simulink model "PARTEB"  (R2020b)
settings: Solver=VariableStepAuto  StartTime=0.0  StopTime=20  RelTol=1e-3
libraries: pid_lib x1
settings Model: Creator=User  LastModifiedBy=angello

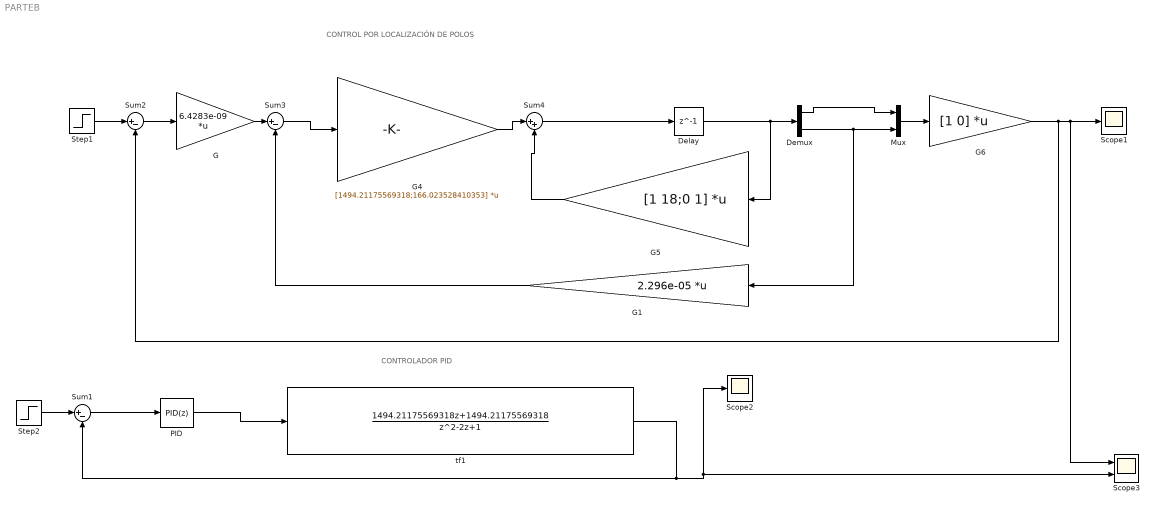
== system PARTEB ==
  note: CONTROL POR LOCALIZACIÓN DE POLOS
  note: CONTROLADOR PID
  Delay : Delay  DelayLength=1  InitialCondition=0
  Demux : Demux  Outputs=2
  G : Gain  Gain=6.4283e-09  Multiplication=Matrix(K*u)
  G1 : Gain  Gain=2.296e-05  Multiplication=Matrix(K*u)
  G4 : Gain  Gain=[1494.21175569318;166.023528410353]  Multiplication=Matrix(K*u)
  G5 : Gain  Gain=[1 18;0 1]  Multiplication=Matrix(K*u)
  G6 : Gain  Gain=[1 0]  Multiplication=Matrix(K*u)
  Mux : Mux  Inputs=2
  PID : pid_lib/PID Controller  Controller=PID  Form=Parallel  TimeDomain=Discrete-time  UseExternalTs=off  SampleTime=-1  IntegratorMethod=Forward Euler  FilterMethod=Forward Euler  ControllerParametersSource=internal  P=4.3719  I=1.7458  D=10.8844  UseFilter=on  N=100  TunerSelectOption=Transfer Function Based (PID Tuner App)  InitialConditionSource=internal  InitialConditionForIntegrator=0  InitialConditionForFilter=0  DifferentiatorICPrevScaledInput=0  ExternalReset=none  TrackingMode=off  Kt=1  LimitOutput=off  SatLimitsSource=internal  UpperSaturationLimit=inf  LowerSaturationLimit=-inf  LinearizeAsGain=off  AntiWindupMode=none  Kb=1  POutMin=[]  POutMax=[]  IOutMin=[]  IOutMax=[]  DOutMin=[]  DOutMax=[]  NOutMin=[]  NOutMax=[]  SumOutMin=[]  SumOutMax=[]  SaturationOutMin=[]  SaturationOutMax=[]  PParamMin=[]  PParamMax=[]  IParamMin=[]  IParamMax=[]  DParamMin=[]  DParamMax=[]  NParamMin=[]  NParamMax=[]  KbParamMin=[]  KbParamMax=[]  KtParamMin=[]  KtParamMax=[]  KbOutMin=[]  KbOutMax=[]  KtOutMin=[]  KtOutMax=[]  IntegratorOutMin=[]  IntegratorOutMax=[]  FilterOutMin=[]  FilterOutMax=[]  SumI1OutMin=[]  SumI1OutMax=[]  SumI2OutMin=[]  SumI2OutMax=[]  SumI3OutMin=[]  SumI3OutMax=[]  SumI4OutMin=[]  SumI4OutMax=[]  SumDOutMin=[]  SumDOutMax=[]  DifferentiatorOutMin=[]  DifferentiatorOutMax=[]  FilterDiffOutCoefMin=[]  FilterDiffOutCoefMax=[]  ReciprocalOutMin=[]  ReciprocalOutMax=[]  SumDenOutMin=[]  SumDenOutMax=[]  SumNumOutMin=[]  SumNumOutMax=[]  DivideOutMin=[]  DivideOutMax=[]  UdiffTsProdOutMin=[]  UdiffTsProdOutMax=[]  NTsProdOutMin=[]  NTsProdOutMax=[]  UintegralTsProdOutMin=[]  UintegralTsProdOutMax=[]  UngainTsProdOutMin=[]  UngainTsProdOutMax=[]  IntegratorContinuousStateAttributes=''  IntegratorStateMustResolveToSignalObject=off  IntegratorRTWStateStorageClass=Auto  FilterContinuousStateAttributes=''  FilterStateMustResolveToSignalObject=off  FilterRTWStateStorageClass=Auto  ParallelPVariant=InternalParameters  IdealPVariant=Disabled  IVariant=InternalParameters  DVariant=InternalParameters  IntegratorVariant=Discrete  SatVariant=Disabled  AWVariant=Passthrough  PCopyVariant=Disabled  TRVariant=Disabled  FdbkBlocksVariant=Forward  IdealPFdbkVariant=Disabled  SatFdbkVariant=Disabled  DerivativeFilterVariant=ForwardEulerFilter  NVariant=InternalParameters  NCopyVariant=Disabled  FilterICVariant=InternalICsFilter  IntegratorICVariant=InternalICs  ExternalResetVariant=Disabled  TRSumVariant=Passthrough  SumFdbkVariant=Disabled  SumVariant=Sum_PID  TsampFilterVariant=InternalTs  TsampNgainVariant=Passthrough  TsampIntegralVariant=Passthrough  ExternalSaturationOutDataTypeStr=Inherit: Same as second input
  Scope1 : Scope
  Scope2 : Scope
  Scope3 : Scope  NumInputPorts=2
  Step1 : Step  Time=0  SampleTime=0.01
  Step2 : Step  Time=0  SampleTime=0.01
  Sum1 : Sum  Inputs=|+-
  Sum2 : Sum  Inputs=|+-
  Sum3 : Sum  Inputs=|+-
  Sum4 : Sum  Inputs=|++
  tf1 : DiscreteTransferFcn  Numerator=[0 1494.21175569318 1494.21175569318]  Denominator=[1 -2 1]
  wires:
  Delay/1 -> G5/1, Demux/1
  Sum2/1 -> G/1
  G/1 -> Sum3/1
  Step1/1 -> Sum2/1
  G1/1 -> Sum3/2
  Sum3/1 -> G4/1
  G4/1 -> Sum4/1
  G5/1 -> Sum4/2
  Sum4/1 -> Delay/1
  G6/1 -> Scope3/1, Scope1/1, Sum2/2
  Mux/1 -> G6/1
  Demux/2 -> Mux/2, G1/1
  Demux/1 -> Mux/1
  tf1/1 -> Scope3/2, Scope2/1, Sum1/2
  Step2/1 -> Sum1/1
  PID/1 -> tf1/1
  Sum1/1 -> PID/1
